simulink model "Scenario_13_CoDeSys"  (R2012b)
settings: Solver=ode3  StartTime=0.0  StopTime=inf  FixedStep=Sample_Time_Model  RelTol=1e-3
PreLoadFcn:
  | Variablen_Scenario13
InitFcn:
  | BT = randperm(9);
values from neighbouring files (symbols this model uses):
  Band_Geschwindigkeit = 1.47    [Variablen_Scenario13.m]
  Band_Sensor_Hell_2_Z = -6.5    [Variablen_Scenario13.m]
  Band_Sensor_Hell_3_Z = -10.36    [Variablen_Scenario13.m]
  Band_Sensor_Hell_4_Z = -14.64    [Variablen_Scenario13.m]
  Band_Sensor_Tolerance_Z = 0.2    [Variablen_Scenario13.m]
  Bauteil_Fallgeschwindigkeit = 0.4    [Variablen_Scenario13.m]
  Bauteil_Farbe_Metall = [0.8 0.8 0.8]    [Variablen_Scenario13.m]
  Bauteil_Farbe_Schwarz = [0.2 0.2 0.2]    [Variablen_Scenario13.m]
  Bauteil_Farbe_Weiss = [1 1 0.2]    [Variablen_Scenario13.m]
  Kran_Dauer_90_Grad = 5    [Variablen_Scenario13.m]
  Kran_Drehwinkel_90_Grad = 8050    [Variablen_Scenario13.m]
  Kran_Sensor_Position_Delta = 0.07    [Variablen_Scenario13.m]
  Sample_Time_Model = 0.05    [Variablen_Scenario13.m]
  Sample_Time_Simulation = 0.1    [Variablen_Scenario13.m]
  Sensor_Band_Metall_1 = -6.5    [Variablen_Scenario13.m]
  Sensor_Band_Metall_2 = -10.36    [Variablen_Scenario13.m]
libraries: simulink x557, vrlib x13, opclib x7, rtwinlib x1
(part 8 of 10)

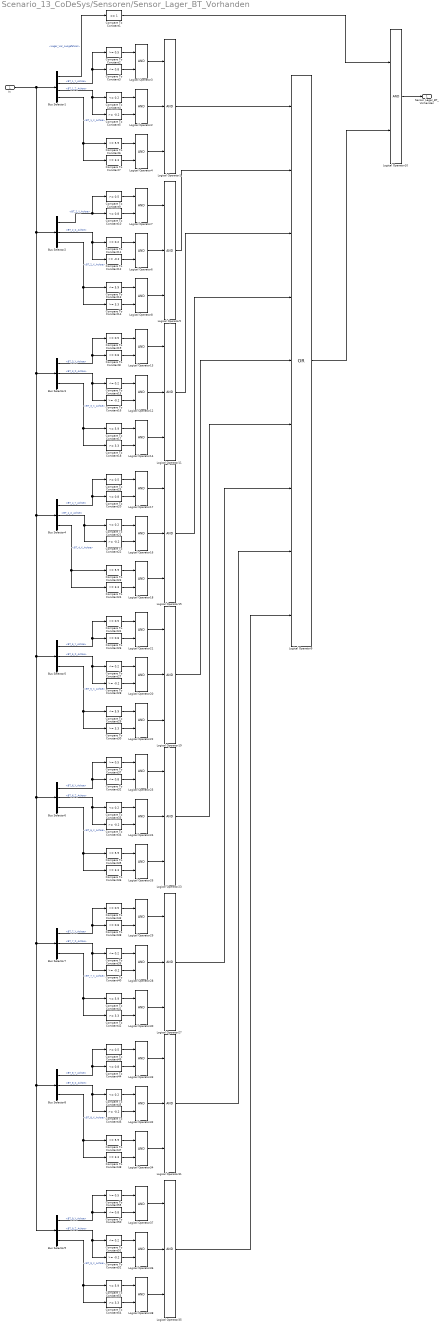
== system Scenario_13_CoDeSys/Sensoren/Sensor_Lager_BT_Vorhanden ==
  In : Inport
  Bus Selector1 : BusSelector  OutputSignals=Bauteil.Stempelanlage_BT.Stempelanlage.Lager.Lager_Ver_Ausgefahren,Bauteil.Stempelanlage_BT.Bauteil_1.BT_1_Y_Achse,Bauteil.Stempelanlage_BT.Bauteil_1.BT_1_Z_Achse,Bauteil.Stempelanlage_BT.Bauteil_1.BT_1_X_Achse
  Bus Selector2 : BusSelector  OutputSignals=Bauteil.Stempelanlage_BT.Bauteil_2.BT_2_Y_Achse,Bauteil.Stempelanlage_BT.Bauteil_2.BT_2_Z_Achse,Bauteil.Stempelanlage_BT.Bauteil_2.BT_2_X_Achse
  Bus Selector3 : BusSelector  OutputSignals=Bauteil.Stempelanlage_BT.Bauteil_3.BT_3_Y_Achse,Bauteil.Stempelanlage_BT.Bauteil_3.BT_3_Z_Achse,Bauteil.Stempelanlage_BT.Bauteil_3.BT_3_X_Achse
  Bus Selector4 : BusSelector  OutputSignals=Bauteil.Stempelanlage_BT.Bauteil_4.BT_4_Y_Achse,Bauteil.Stempelanlage_BT.Bauteil_4.BT_4_Z_Achse,Bauteil.Stempelanlage_BT.Bauteil_4.BT_4_X_Achse
  Bus Selector5 : BusSelector  OutputSignals=Bauteil.Stempelanlage_BT.Bauteil_5.BT_5_Y_Achse,Bauteil.Stempelanlage_BT.Bauteil_5.BT_5_Z_Achse,Bauteil.Stempelanlage_BT.Bauteil_5.BT_5_X_Achse
  Bus Selector6 : BusSelector  OutputSignals=Bauteil.Stempelanlage_BT.Bauteil_6.BT_6_Y_Achse,Bauteil.Stempelanlage_BT.Bauteil_6.BT_6_Z_Achse,Bauteil.Stempelanlage_BT.Bauteil_6.BT_6_X_Achse
  Bus Selector7 : BusSelector  OutputSignals=Bauteil.Stempelanlage_BT.Bauteil_7.BT_7_Y_Achse,Bauteil.Stempelanlage_BT.Bauteil_7.BT_7_Z_Achse,Bauteil.Stempelanlage_BT.Bauteil_7.BT_7_X_Achse
  Bus Selector8 : BusSelector  OutputSignals=Bauteil.Stempelanlage_BT.Bauteil_8.BT_8_Y_Achse,Bauteil.Stempelanlage_BT.Bauteil_8.BT_8_Z_Achse,Bauteil.Stempelanlage_BT.Bauteil_8.BT_8_X_Achse
  Bus Selector9 : BusSelector  OutputSignals=Bauteil.Stempelanlage_BT.Bauteil_9.BT_9_Y_Achse,Bauteil.Stempelanlage_BT.Bauteil_9.BT_9_Z_Achse,Bauteil.Stempelanlage_BT.Bauteil_9.BT_9_X_Achse
  Compare To Constant1 : simulink/Logic and Bit Operations/Compare To Constant  relop===  const=1  OutDataTypeStr=boolean
  Compare To Constant{3,8,10,20,26,32,38,44,50} (9 alike) : simulink/Logic and Bit Operations/Compare To Constant  relop=<=  const=0.8  OutDataTypeStr=boolean
  Compare To Constant{4,11,15,21,27,33,39,45,51} (9 alike) : simulink/Logic and Bit Operations/Compare To Constant  relop=<=  const=0.2  OutDataTypeStr=boolean
  Compare To Constant{5,12,16,22,28,34,40,46,52} (9 alike) : simulink/Logic and Bit Operations/Compare To Constant  relop=>=  const=-0.2  OutDataTypeStr=boolean
  Compare To Constant{6,13,17,23,29,35,41,47,53} (9 alike) : simulink/Logic and Bit Operations/Compare To Constant  relop=<=  const=5.9  OutDataTypeStr=boolean
  Compare To Constant{7,14,18,24,30,36,42,48,54} (9 alike) : simulink/Logic and Bit Operations/Compare To Constant  relop=>=  const=3.3  OutDataTypeStr=boolean
  Compare To Constant{2,9,19,25,31,37,43,49,55} (9 alike) : simulink/Logic and Bit Operations/Compare To Constant  relop=>=  const=0.5  OutDataTypeStr=boolean
  Logical Operator{1,5,11,15,19,23,27,31,35} (9 alike) : Logic  Inputs=3  AllPortsSameDT=off  OutDataTypeStr=boolean
  Logical Operator{2..4,6..8,10,12..14,16..18,20..22,24..26,28..30,32..34,36..38} (28 alike) : Logic  AllPortsSameDT=off  OutDataTypeStr=boolean
  Logical Operator9 : Logic  Operator=OR  Inputs=9  AllPortsSameDT=off  OutDataTypeStr=boolean
  Sensor_Lager_BT_Vorhanden : Outport
  wires:
  Compare To Constant2/1 -> Logical Operator3/1
  Compare To Constant3/1 -> Logical Operator3/2
  Compare To Constant1/1 -> Logical Operator10/1
  Logical Operator3/1 -> Logical Operator1/1
  Compare To Constant4/1 -> Logical Operator2/1
  Compare To Constant5/1 -> Logical Operator2/2
  Logical Operator2/1 -> Logical Operator1/2
  Compare To Constant6/1 -> Logical Operator4/1
  Compare To Constant7/1 -> Logical Operator4/2
  Logical Operator4/1 -> Logical Operator1/3
  Bus Selector1/1 -> Compare To Constant1/1  "<Lager_Ver_Ausgefahren>"
  Bus Selector1/2 -> Compare To Constant2/1, Compare To Constant3/1  "<BT_1_Y_Achse>"
  Bus Selector1/3 -> Compare To Constant4/1, Compare To Constant5/1  "<BT_1_Z_Achse>"
  Bus Selector1/4 -> Compare To Constant6/1, Compare To Constant7/1  "<BT_1_X_Achse>"
  Compare To Constant9/1 -> Logical Operator7/1
  Compare To Constant10/1 -> Logical Operator7/2
  Logical Operator7/1 -> Logical Operator5/1
  Logical Operator5/1 -> Logical Operator9/2
  Compare To Constant11/1 -> Logical Operator6/1
  Compare To Constant12/1 -> Logical Operator6/2
  Logical Operator6/1 -> Logical Operator5/2
  Compare To Constant13/1 -> Logical Operator8/1
  Compare To Constant14/1 -> Logical Operator8/2
  Logical Operator8/1 -> Logical Operator5/3
  Bus Selector2/1 -> Compare To Constant9/1, Compare To Constant10/1  "<BT_2_Y_Achse>"
  Bus Selector2/2 -> Compare To Constant11/1, Compare To Constant12/1  "<BT_2_Z_Achse>"
  Bus Selector2/3 -> Compare To Constant13/1, Compare To Constant14/1  "<BT_2_X_Achse>"
  Logical Operator9/1 -> Logical Operator10/2
  Logical Operator10/1 -> Sensor_Lager_BT_Vorhanden/1
  Logical Operator1/1 -> Logical Operator9/1
  Compare To Constant19/1 -> Logical Operator13/1
  Compare To Constant8/1 -> Logical Operator13/2
  Logical Operator13/1 -> Logical Operator11/1
  Compare To Constant15/1 -> Logical Operator12/1
  Compare To Constant16/1 -> Logical Operator12/2
  Logical Operator12/1 -> Logical Operator11/2
  Compare To Constant17/1 -> Logical Operator14/1
  Compare To Constant18/1 -> Logical Operator14/2
  Logical Operator14/1 -> Logical Operator11/3
  Bus Selector3/1 -> Compare To Constant19/1, Compare To Constant8/1  "<BT_3_Y_Achse>"
  Bus Selector3/2 -> Compare To Constant15/1, Compare To Constant16/1  "<BT_3_Z_Achse>"
  Bus Selector3/3 -> Compare To Constant17/1, Compare To Constant18/1  "<BT_3_X_Achse>"
  Compare To Constant25/1 -> Logical Operator17/1
  Compare To Constant20/1 -> Logical Operator17/2
  Logical Operator17/1 -> Logical Operator15/1
  Compare To Constant21/1 -> Logical Operator16/1
  Compare To Constant22/1 -> Logical Operator16/2
  Logical Operator16/1 -> Logical Operator15/2
  Compare To Constant23/1 -> Logical Operator18/1
  Compare To Constant24/1 -> Logical Operator18/2
  Logical Operator18/1 -> Logical Operator15/3
  Bus Selector4/1 -> Compare To Constant25/1, Compare To Constant20/1  "<BT_4_Y_Achse>"
  Compare To Constant31/1 -> Logical Operator21/1
  Compare To Constant26/1 -> Logical Operator21/2
  Logical Operator21/1 -> Logical Operator19/1
  Compare To Constant27/1 -> Logical Operator20/1
  Compare To Constant28/1 -> Logical Operator20/2
  Logical Operator20/1 -> Logical Operator19/2
  Compare To Constant29/1 -> Logical Operator22/1
  Compare To Constant30/1 -> Logical Operator22/2
  Logical Operator22/1 -> Logical Operator19/3
  Bus Selector5/1 -> Compare To Constant31/1, Compare To Constant26/1  "<BT_5_Y_Achse>"
  Bus Selector5/2 -> Compare To Constant27/1, Compare To Constant28/1  "<BT_5_Z_Achse>"
  Bus Selector5/3 -> Compare To Constant29/1, Compare To Constant30/1  "<BT_5_X_Achse>"
  Compare To Constant37/1 -> Logical Operator25/1
  Compare To Constant32/1 -> Logical Operator25/2
  Logical Operator25/1 -> Logical Operator23/1
  Compare To Constant33/1 -> Logical Operator24/1
  Compare To Constant34/1 -> Logical Operator24/2
  Logical Operator24/1 -> Logical Operator23/2
  Compare To Constant35/1 -> Logical Operator26/1
  Compare To Constant36/1 -> Logical Operator26/2
  Logical Operator26/1 -> Logical Operator23/3
  Bus Selector6/1 -> Compare To Constant37/1, Compare To Constant32/1  "<BT_6_Y_Achse>"
  Bus Selector6/2 -> Compare To Constant33/1, Compare To Constant34/1  "<BT_6_Z_Achse>"
  Bus Selector6/3 -> Compare To Constant35/1, Compare To Constant36/1  "<BT_6_X_Achse>"
  Logical Operator11/1 -> Logical Operator9/3
  Logical Operator15/1 -> Logical Operator9/4
  Logical Operator19/1 -> Logical Operator9/5
  Logical Operator23/1 -> Logical Operator9/6
  Bus Selector4/2 -> Compare To Constant21/1, Compare To Constant22/1  "<BT_4_Z_Achse>"
  Bus Selector4/3 -> Compare To Constant23/1, Compare To Constant24/1  "<BT_4_X_Achse>"
  Compare To Constant43/1 -> Logical Operator29/1
  Compare To Constant38/1 -> Logical Operator29/2
  Logical Operator29/1 -> Logical Operator27/1
  Compare To Constant39/1 -> Logical Operator28/1
  Compare To Constant40/1 -> Logical Operator28/2
  Logical Operator28/1 -> Logical Operator27/2
  Compare To Constant41/1 -> Logical Operator30/1
  Compare To Constant42/1 -> Logical Operator30/2
  Logical Operator30/1 -> Logical Operator27/3
  Bus Selector7/1 -> Compare To Constant43/1, Compare To Constant38/1  "<BT_7_Y_Achse>"
  Bus Selector7/2 -> Compare To Constant39/1, Compare To Constant40/1  "<BT_7_Z_Achse>"
  Bus Selector7/3 -> Compare To Constant41/1, Compare To Constant42/1  "<BT_7_X_Achse>"
  Compare To Constant49/1 -> Logical Operator33/1
  Compare To Constant44/1 -> Logical Operator33/2
  Logical Operator33/1 -> Logical Operator31/1
  Compare To Constant45/1 -> Logical Operator32/1
  Compare To Constant46/1 -> Logical Operator32/2
  Logical Operator32/1 -> Logical Operator31/2
  Compare To Constant47/1 -> Logical Operator34/1
  Compare To Constant48/1 -> Logical Operator34/2
  Logical Operator34/1 -> Logical Operator31/3
  Bus Selector8/1 -> Compare To Constant49/1, Compare To Constant44/1  "<BT_8_Y_Achse>"
  Bus Selector8/2 -> Compare To Constant45/1, Compare To Constant46/1  "<BT_8_Z_Achse>"
  Bus Selector8/3 -> Compare To Constant47/1, Compare To Constant48/1  "<BT_8_X_Achse>"
  Compare To Constant55/1 -> Logical Operator37/1
  Compare To Constant50/1 -> Logical Operator37/2
  Logical Operator37/1 -> Logical Operator35/1
  Compare To Constant51/1 -> Logical Operator36/1
  Compare To Constant52/1 -> Logical Operator36/2
  Logical Operator36/1 -> Logical Operator35/2
  Compare To Constant53/1 -> Logical Operator38/1
  Compare To Constant54/1 -> Logical Operator38/2
  Logical Operator38/1 -> Logical Operator35/3
  In/1 -> Bus Selector2/1, Bus Selector4/1, Bus Selector6/1, Bus Selector9/1, Bus Selector8/1, Bus Selector7/1, Bus Selector5/1, Bus Selector3/1, Bus Selector1/1
  Bus Selector9/1 -> Compare To Constant55/1, Compare To Constant50/1  "<BT_9_Y_Achse>"
  Bus Selector9/2 -> Compare To Constant51/1, Compare To Constant52/1  "<BT_9_Z_Achse>"
  Bus Selector9/3 -> Compare To Constant53/1, Compare To Constant54/1  "<BT_9_X_Achse>"
  Logical Operator35/1 -> Logical Operator9/9
  Logical Operator31/1 -> Logical Operator9/8
  Logical Operator27/1 -> Logical Operator9/7

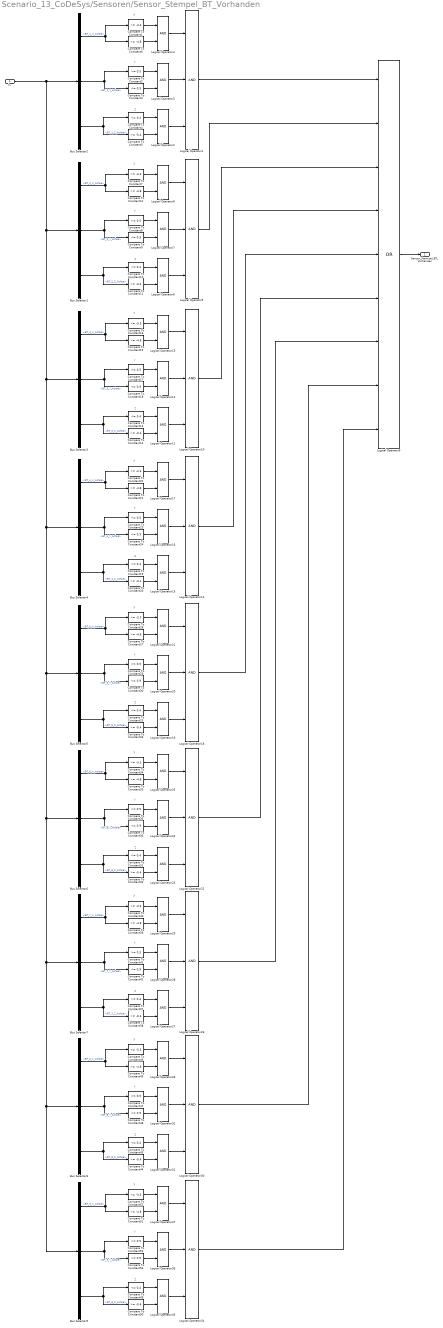
== system Scenario_13_CoDeSys/Sensoren/Sensor_Stempel_BT_Vorhanden ==
  note: Z
  note: Y
  note: X
  note: Z
  note: Y
  note: X
  note: Z
  note: Y
  note: X
  note: Z
  note: Y
  note: X
  note: Z
  note: Y
  note: X
  note: Z
  note: Y
  note: X
  note: Z
  note: Y
  note: X
  note: Z
  note: Y
  note: X
  note: Z
  note: Y
  note: X
  In : Inport
  Bus Selector1 : BusSelector  OutputSignals=Bauteil.Stempelanlage_BT.Bauteil_2.BT_2_X_Achse,Bauteil.Stempelanlage_BT.Bauteil_2.BT_2_Y_Achse,Bauteil.Stempelanlage_BT.Bauteil_2.BT_2_Z_Achse
  Bus Selector2 : BusSelector  OutputSignals=Bauteil.Stempelanlage_BT.Bauteil_1.BT_1_X_Achse,Bauteil.Stempelanlage_BT.Bauteil_1.BT_1_Y_Achse,Bauteil.Stempelanlage_BT.Bauteil_1.BT_1_Z_Achse
  Bus Selector3 : BusSelector  OutputSignals=Bauteil.Stempelanlage_BT.Bauteil_3.BT_3_X_Achse,Bauteil.Stempelanlage_BT.Bauteil_3.BT_3_Y_Achse,Bauteil.Stempelanlage_BT.Bauteil_3.BT_3_Z_Achse
  Bus Selector4 : BusSelector  OutputSignals=Bauteil.Stempelanlage_BT.Bauteil_4.BT_4_X_Achse,Bauteil.Stempelanlage_BT.Bauteil_4.BT_4_Y_Achse,Bauteil.Stempelanlage_BT.Bauteil_4.BT_4_Z_Achse
  Bus Selector5 : BusSelector  OutputSignals=Bauteil.Stempelanlage_BT.Bauteil_5.BT_5_X_Achse,Bauteil.Stempelanlage_BT.Bauteil_5.BT_5_Y_Achse,Bauteil.Stempelanlage_BT.Bauteil_5.BT_5_Z_Achse
  Bus Selector6 : BusSelector  OutputSignals=Bauteil.Stempelanlage_BT.Bauteil_6.BT_6_X_Achse,Bauteil.Stempelanlage_BT.Bauteil_6.BT_6_Y_Achse,Bauteil.Stempelanlage_BT.Bauteil_6.BT_6_Z_Achse
  Bus Selector7 : BusSelector  OutputSignals=Bauteil.Stempelanlage_BT.Bauteil_7.BT_7_X_Achse,Bauteil.Stempelanlage_BT.Bauteil_7.BT_7_Y_Achse,Bauteil.Stempelanlage_BT.Bauteil_7.BT_7_Z_Achse
  Bus Selector8 : BusSelector  OutputSignals=Bauteil.Stempelanlage_BT.Bauteil_8.BT_8_X_Achse,Bauteil.Stempelanlage_BT.Bauteil_8.BT_8_Y_Achse,Bauteil.Stempelanlage_BT.Bauteil_8.BT_8_Z_Achse
  Bus Selector9 : BusSelector  OutputSignals=Bauteil.Stempelanlage_BT.Bauteil_9.BT_9_X_Achse,Bauteil.Stempelanlage_BT.Bauteil_9.BT_9_Y_Achse,Bauteil.Stempelanlage_BT.Bauteil_9.BT_9_Z_Achse
  Compare To Constant{1,7,16,22,28,34,40,46,52} (9 alike) : simulink/Logic and Bit Operations/Compare To Constant  relop=<=  const=-3.3  OutDataTypeStr=boolean
  Compare To Constant{4,10,13,19,25,31,37,43,49} (9 alike) : simulink/Logic and Bit Operations/Compare To Constant  relop=<=  const=0.4  OutDataTypeStr=boolean
  Compare To Constant{5,11,14,20,26,32,38,44,50} (9 alike) : simulink/Logic and Bit Operations/Compare To Constant  relop=>=  const=-0.4  OutDataTypeStr=boolean
  Compare To Constant{6,12,15,21,27,33,39,45,51} (9 alike) : simulink/Logic and Bit Operations/Compare To Constant  relop=>=  const=-4.8  OutDataTypeStr=boolean
  Compare To Constant{2,8,17,23,29,35,41,47,53} (9 alike) : simulink/Logic and Bit Operations/Compare To Constant  relop=>=  const=0.5  OutDataTypeStr=boolean
  Compare To Constant{3,9,18,24,30,36,42,48,54} (9 alike) : simulink/Logic and Bit Operations/Compare To Constant  relop=<=  const=0.9  OutDataTypeStr=boolean
  Logical Operator{1,5,10,14,18,22,26,30,34} (9 alike) : Logic  Inputs=3  AllPortsSameDT=off  OutDataTypeStr=boolean
  Logical Operator{2..4,6..8,11..13,15..17,19..21,23..25,27..29,31..33,35..37} (27 alike) : Logic  AllPortsSameDT=off  OutDataTypeStr=boolean
  Logical Operator9 : Logic  Operator=OR  Inputs=9  AllPortsSameDT=off  OutDataTypeStr=boolean
  Sensor_Stempel_BT_Vorhanden : Outport
  wires:
  Compare To Constant2/1 -> Logical Operator3/1
  Compare To Constant3/1 -> Logical Operator3/2
  Logical Operator3/1 -> Logical Operator1/2
  Compare To Constant4/1 -> Logical Operator2/1
  Compare To Constant5/1 -> Logical Operator2/2
  Logical Operator2/1 -> Logical Operator1/3
  Compare To Constant1/1 -> Logical Operator4/1
  Compare To Constant6/1 -> Logical Operator4/2
  Logical Operator4/1 -> Logical Operator1/1
  Bus Selector2/1 -> Compare To Constant6/1, Compare To Constant1/1  "<BT_1_X_Achse>"
  Bus Selector2/2 -> Compare To Constant3/1, Compare To Constant2/1  "<BT_1_Y_Achse>"
  Bus Selector2/3 -> Compare To Constant5/1, Compare To Constant4/1  "<BT_1_Z_Achse>"
  Compare To Constant8/1 -> Logical Operator7/1
  Compare To Constant9/1 -> Logical Operator7/2
  Logical Operator7/1 -> Logical Operator5/2
  Compare To Constant10/1 -> Logical Operator6/1
  Compare To Constant11/1 -> Logical Operator6/2
  Logical Operator6/1 -> Logical Operator5/3
  Compare To Constant7/1 -> Logical Operator8/1
  Compare To Constant12/1 -> Logical Operator8/2
  Logical Operator8/1 -> Logical Operator5/1
  Bus Selector1/1 -> Compare To Constant12/1, Compare To Constant7/1  "<BT_2_X_Achse>"
  Bus Selector1/2 -> Compare To Constant9/1, Compare To Constant8/1  "<BT_2_Y_Achse>"
  Bus Selector1/3 -> Compare To Constant11/1, Compare To Constant10/1  "<BT_2_Z_Achse>"
  Logical Operator1/1 -> Logical Operator9/1
  Logical Operator5/1 -> Logical Operator9/2
  Logical Operator9/1 -> Sensor_Stempel_BT_Vorhanden/1
  Compare To Constant17/1 -> Logical Operator12/1
  Compare To Constant18/1 -> Logical Operator12/2
  Logical Operator12/1 -> Logical Operator10/2
  Compare To Constant13/1 -> Logical Operator11/1
  Compare To Constant14/1 -> Logical Operator11/2
  Logical Operator11/1 -> Logical Operator10/3
  Compare To Constant16/1 -> Logical Operator13/1
  Compare To Constant15/1 -> Logical Operator13/2
  Logical Operator13/1 -> Logical Operator10/1
  Bus Selector3/1 -> Compare To Constant15/1, Compare To Constant16/1  "<BT_3_X_Achse>"
  Bus Selector3/2 -> Compare To Constant18/1, Compare To Constant17/1  "<BT_3_Y_Achse>"
  Bus Selector3/3 -> Compare To Constant14/1, Compare To Constant13/1  "<BT_3_Z_Achse>"
  Compare To Constant23/1 -> Logical Operator16/1
  Compare To Constant24/1 -> Logical Operator16/2
  Logical Operator16/1 -> Logical Operator14/2
  Compare To Constant19/1 -> Logical Operator15/1
  Compare To Constant20/1 -> Logical Operator15/2
  Logical Operator15/1 -> Logical Operator14/3
  Compare To Constant22/1 -> Logical Operator17/1
  Compare To Constant21/1 -> Logical Operator17/2
  Logical Operator17/1 -> Logical Operator14/1
  Bus Selector4/1 -> Compare To Constant21/1, Compare To Constant22/1  "<BT_4_X_Achse>"
  Bus Selector4/2 -> Compare To Constant24/1, Compare To Constant23/1  "<BT_4_Y_Achse>"
  Bus Selector4/3 -> Compare To Constant20/1, Compare To Constant19/1  "<BT_4_Z_Achse>"
  Compare To Constant29/1 -> Logical Operator20/1
  Compare To Constant30/1 -> Logical Operator20/2
  Logical Operator20/1 -> Logical Operator18/2
  Compare To Constant25/1 -> Logical Operator19/1
  Compare To Constant26/1 -> Logical Operator19/2
  Logical Operator19/1 -> Logical Operator18/3
  Compare To Constant28/1 -> Logical Operator21/1
  Compare To Constant27/1 -> Logical Operator21/2
  Logical Operator21/1 -> Logical Operator18/1
  Bus Selector5/1 -> Compare To Constant27/1, Compare To Constant28/1  "<BT_5_X_Achse>"
  Bus Selector5/2 -> Compare To Constant30/1, Compare To Constant29/1  "<BT_5_Y_Achse>"
  Bus Selector5/3 -> Compare To Constant26/1, Compare To Constant25/1  "<BT_5_Z_Achse>"
  Compare To Constant35/1 -> Logical Operator24/1
  Compare To Constant36/1 -> Logical Operator24/2
  Logical Operator24/1 -> Logical Operator22/2
  Compare To Constant31/1 -> Logical Operator23/1
  Compare To Constant32/1 -> Logical Operator23/2
  Logical Operator23/1 -> Logical Operator22/3
  Compare To Constant34/1 -> Logical Operator25/1
  Compare To Constant33/1 -> Logical Operator25/2
  Logical Operator25/1 -> Logical Operator22/1
  Bus Selector6/1 -> Compare To Constant33/1, Compare To Constant34/1  "<BT_6_X_Achse>"
  Bus Selector6/2 -> Compare To Constant36/1, Compare To Constant35/1  "<BT_6_Y_Achse>"
  Bus Selector6/3 -> Compare To Constant32/1, Compare To Constant31/1  "<BT_6_Z_Achse>"
  Logical Operator10/1 -> Logical Operator9/3
  Logical Operator14/1 -> Logical Operator9/4
  Logical Operator18/1 -> Logical Operator9/5
  Logical Operator22/1 -> Logical Operator9/6
  Compare To Constant41/1 -> Logical Operator28/1
  Compare To Constant42/1 -> Logical Operator28/2
  Logical Operator28/1 -> Logical Operator26/2
  Compare To Constant37/1 -> Logical Operator27/1
  Compare To Constant38/1 -> Logical Operator27/2
  Logical Operator27/1 -> Logical Operator26/3
  Compare To Constant40/1 -> Logical Operator29/1
  Compare To Constant39/1 -> Logical Operator29/2
  Logical Operator29/1 -> Logical Operator26/1
  Bus Selector7/1 -> Compare To Constant39/1, Compare To Constant40/1  "<BT_7_X_Achse>"
  Bus Selector7/2 -> Compare To Constant42/1, Compare To Constant41/1  "<BT_7_Y_Achse>"
  Bus Selector7/3 -> Compare To Constant38/1, Compare To Constant37/1  "<BT_7_Z_Achse>"
  Compare To Constant47/1 -> Logical Operator32/1
  Compare To Constant48/1 -> Logical Operator32/2
  Logical Operator32/1 -> Logical Operator30/2
  Compare To Constant43/1 -> Logical Operator31/1
  Compare To Constant44/1 -> Logical Operator31/2
  Logical Operator31/1 -> Logical Operator30/3
  Compare To Constant46/1 -> Logical Operator33/1
  Compare To Constant45/1 -> Logical Operator33/2
  Logical Operator33/1 -> Logical Operator30/1
  Bus Selector8/1 -> Compare To Constant45/1, Compare To Constant46/1  "<BT_8_X_Achse>"
  Bus Selector8/2 -> Compare To Constant48/1, Compare To Constant47/1  "<BT_8_Y_Achse>"
  Bus Selector8/3 -> Compare To Constant44/1, Compare To Constant43/1  "<BT_8_Z_Achse>"
  Compare To Constant53/1 -> Logical Operator36/1
  Compare To Constant54/1 -> Logical Operator36/2
  Logical Operator36/1 -> Logical Operator34/2
  Compare To Constant49/1 -> Logical Operator35/1
  Compare To Constant50/1 -> Logical Operator35/2
  Logical Operator35/1 -> Logical Operator34/3
  Compare To Constant52/1 -> Logical Operator37/1
  Compare To Constant51/1 -> Logical Operator37/2
  Logical Operator37/1 -> Logical Operator34/1
  In/1 -> Bus Selector1/1, Bus Selector4/1, Bus Selector6/1, Bus Selector7/1, Bus Selector8/1, Bus Selector9/1, Bus Selector5/1, Bus Selector3/1, Bus Selector2/1
  Bus Selector9/1 -> Compare To Constant51/1, Compare To Constant52/1  "<BT_9_X_Achse>"
  Bus Selector9/2 -> Compare To Constant54/1, Compare To Constant53/1  "<BT_9_Y_Achse>"
  Bus Selector9/3 -> Compare To Constant50/1, Compare To Constant49/1  "<BT_9_Z_Achse>"
  Logical Operator26/1 -> Logical Operator9/7
  Logical Operator30/1 -> Logical Operator9/8
  Logical Operator34/1 -> Logical Operator9/9

== system Scenario_13_CoDeSys/Sensoren/Sensoren_Lager_Metall_und_Weiss_Schwarz ==
  In : Inport
  Bus Selector1 : BusSelector  OutputSignals=Eingaenge.Bauteile.BT_Eins,Bauteil.Stempelanlage_BT.Bauteil_1.BT_1_Bereit
  Bus Selector2 : BusSelector  OutputSignals=Eingaenge.Bauteile.BT_Zwei,Bauteil.Stempelanlage_BT.Bauteil_2.BT_2_Bereit
  Bus Selector3 : BusSelector  OutputSignals=Eingaenge.Bauteile.BT_Drei,Bauteil.Stempelanlage_BT.Bauteil_3.BT_3_Bereit
  Bus Selector4 : BusSelector  OutputSignals=Eingaenge.Bauteile.BT_Vier,Bauteil.Stempelanlage_BT.Bauteil_4.BT_4_Bereit
  Bus Selector5 : BusSelector  OutputSignals=Eingaenge.Bauteile.BT_Fuenf,Bauteil.Stempelanlage_BT.Bauteil_5.BT_5_Bereit
  Bus Selector6 : BusSelector  OutputSignals=Eingaenge.Bauteile.BT_Sechs,Bauteil.Stempelanlage_BT.Bauteil_6.BT_6_Bereit
  Bus Selector7 : BusSelector  OutputSignals=Eingaenge.Bauteile.BT_Sieben,Bauteil.Stempelanlage_BT.Bauteil_7.BT_7_Bereit
  Bus Selector8 : BusSelector  OutputSignals=Eingaenge.Bauteile.BT_Acht,Bauteil.Stempelanlage_BT.Bauteil_8.BT_8_Bereit
  Bus Selector9 : BusSelector  OutputSignals=Eingaenge.Bauteile.BT_Neun,Bauteil.Stempelanlage_BT.Bauteil_9.BT_9_Bereit
  Compare To Constant{,1,4,6,8,10,12,14,16} (9 alike) : simulink/Logic and Bit Operations/Compare To Constant  relop===  const=0  OutDataTypeStr=boolean
  Compare To Constant{2..3,5,7,9,11,13,15,17} (9 alike) : simulink/Logic and Bit Operations/Compare To Constant  relop===  const=2  OutDataTypeStr=boolean
  Constant{,1..8} (9 alike) : Constant  Value=3
  Logical Operator{,3..10} (9 alike) : Logic  Operator=OR  AllPortsSameDT=off  OutDataTypeStr=boolean
  Logical Operator1 : Logic  Operator=OR  Inputs=9  AllPortsSameDT=off  OutDataTypeStr=boolean
  Logical Operator2 : Logic  Operator=OR  Inputs=9  AllPortsSameDT=off  OutDataTypeStr=boolean
  Switch{,1..8} (9 alike) : Switch  Threshold=1
  Sensor_Lager_Metall : Outport
  Sensor_Lager_Helligkeit : Outport  Port=2
  wires:
  Compare To Constant2/1 -> Logical Operator2/1, Logical Operator/2
  Compare To Constant/1 -> Logical Operator/1
  Bus Selector1/1 -> Switch/1  "<BT_Eins>"
  Switch/1 -> Compare To Constant2/1, Compare To Constant/1
  Constant/1 -> Switch/3
  Logical Operator/1 -> Logical Operator1/1
  Compare To Constant3/1 -> Logical Operator2/2, Logical Operator3/2
  Compare To Constant1/1 -> Logical Operator3/1
  Switch1/1 -> Compare To Constant3/1, Compare To Constant1/1
  Constant1/1 -> Switch1/3
  Logical Operator3/1 -> Logical Operator1/2
  Compare To Constant5/1 -> Logical Operator2/3, Logical Operator4/2
  Compare To Constant4/1 -> Logical Operator4/1
  Switch2/1 -> Compare To Constant5/1, Compare To Constant4/1
  Constant2/1 -> Switch2/3
  Logical Operator4/1 -> Logical Operator1/3
  Compare To Constant7/1 -> Logical Operator2/4, Logical Operator5/2
  Compare To Constant6/1 -> Logical Operator5/1
  Switch3/1 -> Compare To Constant7/1, Compare To Constant6/1
  Constant3/1 -> Switch3/3
  Logical Operator5/1 -> Logical Operator1/4
  Compare To Constant9/1 -> Logical Operator2/5, Logical Operator6/2
  Compare To Constant8/1 -> Logical Operator6/1
  Switch4/1 -> Compare To Constant9/1, Compare To Constant8/1
  Constant4/1 -> Switch4/3
  Logical Operator6/1 -> Logical Operator1/5
  Compare To Constant11/1 -> Logical Operator2/6, Logical Operator7/2
  Compare To Constant10/1 -> Logical Operator7/1
  Switch5/1 -> Compare To Constant11/1, Compare To Constant10/1
  Constant5/1 -> Switch5/3
  Logical Operator7/1 -> Logical Operator1/6
  Logical Operator2/1 -> Sensor_Lager_Metall/1
  Logical Operator1/1 -> Sensor_Lager_Helligkeit/1
  Bus Selector1/2 -> Switch/2  "<BT_1_Bereit>"
  Bus Selector2/1 -> Switch1/1  "<BT_Zwei>"
  Bus Selector2/2 -> Switch1/2  "<BT_2_Bereit>"
  Bus Selector3/1 -> Switch2/1  "<BT_Drei>"
  Bus Selector3/2 -> Switch2/2  "<BT_3_Bereit>"
  Bus Selector4/1 -> Switch3/1  "<BT_Vier>"
  Bus Selector4/2 -> Switch3/2  "<BT_4_Bereit>"
  Bus Selector5/1 -> Switch4/1  "<BT_Fuenf>"
  Bus Selector5/2 -> Switch4/2  "<BT_5_Bereit>"
  Bus Selector6/1 -> Switch5/1  "<BT_Sechs>"
  Bus Selector6/2 -> Switch5/2  "<BT_6_Bereit>"
  Compare To Constant13/1 -> Logical Operator2/7, Logical Operator8/2
  Compare To Constant12/1 -> Logical Operator8/1
  Switch6/1 -> Compare To Constant13/1, Compare To Constant12/1
  Constant6/1 -> Switch6/3
  Logical Operator8/1 -> Logical Operator1/7
  Bus Selector7/1 -> Switch6/1  "<BT_Sieben>"
  Bus Selector7/2 -> Switch6/2  "<BT_7_Bereit>"
  Compare To Constant15/1 -> Logical Operator2/8, Logical Operator9/2
  Compare To Constant14/1 -> Logical Operator9/1
  Switch7/1 -> Compare To Constant15/1, Compare To Constant14/1
  Constant7/1 -> Switch7/3
  Logical Operator9/1 -> Logical Operator1/8
  Bus Selector8/1 -> Switch7/1  "<BT_Acht>"
  Bus Selector8/2 -> Switch7/2  "<BT_8_Bereit>"
  Compare To Constant17/1 -> Logical Operator2/9, Logical Operator10/2
  Compare To Constant16/1 -> Logical Operator10/1
  Switch8/1 -> Compare To Constant17/1, Compare To Constant16/1
  Constant8/1 -> Switch8/3
  Logical Operator10/1 -> Logical Operator1/9
  In/1 -> Bus Selector2/1, Bus Selector3/1, Bus Selector4/1, Bus Selector7/1, Bus Selector8/1, Bus Selector9/1, Bus Selector6/1, Bus Selector5/1, Bus Selector1/1
  Bus Selector9/1 -> Switch8/1  "<BT_Neun>"
  Bus Selector9/2 -> Switch8/2  "<BT_9_Bereit>"

== system Scenario_13_CoDeSys/Sensoren/Stempel_Druck_Ist ==
  Sensor_Stempel_BT_Vorhanden : Inport
  Stempel_Halterung_Eingefahren : Inport  Port=2
  Stempel_Zyl_Ausgefahren : Inport  Port=3
  Stempel_Druck_Soll : Inport  Port=4
  Constant : Constant  Value=0
  Logical Operator1 : Logic  Inputs=3  AllPortsSameDT=off  OutDataTypeStr=boolean
  Switch : Switch  Threshold=1
  Stempel_Druck_Ist : Outport
  wires:
  Stempel_Halterung_Eingefahren/1 -> Logical Operator1/2
  Sensor_Stempel_BT_Vorhanden/1 -> Logical Operator1/1
  Stempel_Zyl_Ausgefahren/1 -> Logical Operator1/3
  Logical Operator1/1 -> Switch/2
  Switch/1 -> Stempel_Druck_Ist/1
  Stempel_Druck_Soll/1 -> Switch/1
  Constant/1 -> Switch/3

== system Scenario_13_CoDeSys/Signal Expander/BT_Lager_Status ==
  BT_1_Lager_Position : Inport
  BT_2_Lager_Position : Inport  Port=2
  BT_3_Lager_Position : Inport  Port=3
  BT_4_Lager_Position : Inport  Port=4
  BT_5_Lager_Position : Inport  Port=5
  BT_6_Lager_Position : Inport  Port=6
  BT_7_Lager_Position : Inport  Port=7
  BT_8_Lager_Position : Inport  Port=8
  BT_9_Lager_Position : Inport  Port=9
  Add : Sum  Inputs=+++++++++
  Add1 : Sum  Inputs=+++++++++
  Add2 : Sum  Inputs=+++++++++
  Compare To Constant{1..2,5,8,11,14,17,20,23} (9 alike) : simulink/Logic and Bit Operations/Compare To Constant  relop===  const=1  OutDataTypeStr=boolean
  Compare To Constant{3,6,10,12,15,18,21,24,26} (9 alike) : simulink/Logic and Bit Operations/Compare To Constant  relop===  const=3  OutDataTypeStr=boolean
  Compare To Constant{4,7,9,13,16,19,22,25,27} (9 alike) : simulink/Logic and Bit Operations/Compare To Constant  relop===  const=2  OutDataTypeStr=boolean
  Lager_1_Status : Outport
  Lager_2_Status : Outport  Port=2
  Lager_3_Status : Outport  Port=3
  wires:
  BT_1_Lager_Position/1 -> Compare To Constant10/1, Compare To Constant9/1, Compare To Constant1/1
  BT_2_Lager_Position/1 -> Compare To Constant12/1, Compare To Constant13/1, Compare To Constant11/1
  BT_3_Lager_Position/1 -> Compare To Constant15/1, Compare To Constant16/1, Compare To Constant14/1
  BT_4_Lager_Position/1 -> Compare To Constant18/1, Compare To Constant19/1, Compare To Constant17/1
  BT_5_Lager_Position/1 -> Compare To Constant21/1, Compare To Constant22/1, Compare To Constant20/1
  BT_6_Lager_Position/1 -> Compare To Constant24/1, Compare To Constant25/1, Compare To Constant23/1
  Compare To Constant1/1 -> Add/1
  Compare To Constant11/1 -> Add/2
  Compare To Constant14/1 -> Add/3
  Compare To Constant17/1 -> Add/4
  Compare To Constant20/1 -> Add/5
  Compare To Constant23/1 -> Add/6
  Compare To Constant9/1 -> Add1/1
  Compare To Constant13/1 -> Add1/2
  Compare To Constant16/1 -> Add1/3
  Compare To Constant19/1 -> Add1/4
  Compare To Constant22/1 -> Add1/5
  Compare To Constant25/1 -> Add1/6
  Compare To Constant24/1 -> Add2/6
  Compare To Constant21/1 -> Add2/5
  Compare To Constant18/1 -> Add2/4
  Compare To Constant15/1 -> Add2/3
  Compare To Constant12/1 -> Add2/2
  Compare To Constant10/1 -> Add2/1
  Add/1 -> Lager_1_Status/1
  Add1/1 -> Lager_2_Status/1
  Add2/1 -> Lager_3_Status/1
  BT_7_Lager_Position/1 -> Compare To Constant3/1, Compare To Constant4/1, Compare To Constant2/1
  BT_8_Lager_Position/1 -> Compare To Constant6/1, Compare To Constant7/1, Compare To Constant5/1
  BT_9_Lager_Position/1 -> Compare To Constant26/1, Compare To Constant27/1, Compare To Constant8/1
  Compare To Constant2/1 -> Add/7
  Compare To Constant5/1 -> Add/8
  Compare To Constant8/1 -> Add/9
  Compare To Constant4/1 -> Add1/7
  Compare To Constant7/1 -> Add1/8
  Compare To Constant27/1 -> Add1/9
  Compare To Constant3/1 -> Add2/7
  Compare To Constant6/1 -> Add2/8
  Compare To Constant26/1 -> Add2/9

== system Scenario_13_CoDeSys/Signal Expander/Berechne Band Geschwindigkeit ==
  Constant : Constant  Value=Band_Geschwindigkeit
  Multi : Product  Inputs=**
  Sample_Time : Constant  Value=Sample_Time_Model
  Band_Geschwindigkeit : Outport
  wires:
  Sample_Time/1 -> Multi/2
  Constant/1 -> Multi/1
  Multi/1 -> Band_Geschwindigkeit/1

== system Scenario_13_CoDeSys/Signal Expander/Kran_Position_Sensor ==
  In : Inport
  Abs : Abs
  Add : Sum
  Add1 : Sum  Inputs=+-
  Add2 : Sum
  Add3 : Sum  Inputs=+-
  Constant{,1,3..4,6} (5 alike) : Constant  Value=Kran_Sensor_Position_Delta
  Constant2 : Constant  Value=3.1416
  Constant5 : Constant  Value=1.5708
  Logical Operator1 : Logic  AllPortsSameDT=off  OutDataTypeStr=boolean
  Logical Operator2 : Logic  AllPortsSameDT=off  OutDataTypeStr=boolean
  Relational Operator : RelationalOperator  OutDataTypeStr=boolean
  Relational Operator{1..4} (4 alike) : RelationalOperator  Operator=<=  OutDataTypeStr=boolean
  Sensor_Kran_Stellung_Lager : Outport
  Sensor_Kran_Stellung_Band : Outport  Port=2
  Sensor_Kran_Stellung_Stempel : Outport  Port=3
  wires:
  Constant/1 -> Relational Operator/1
  Abs/1 -> Relational Operator/2
  Relational Operator/1 -> Sensor_Kran_Stellung_Lager/1
  Constant1/1 -> Add/1
  Constant2/1 -> Add1/1, Add/2
  Constant3/1 -> Add1/2
  Add/1 -> Relational Operator1/2
  Add1/1 -> Relational Operator2/1
  Relational Operator1/1 -> Logical Operator1/1
  Relational Operator2/1 -> Logical Operator1/2
  Logical Operator1/1 -> Sensor_Kran_Stellung_Stempel/1
  In/1 -> Relational Operator4/2, Relational Operator3/1, Relational Operator2/2, Relational Operator1/1, Abs/1
  Constant4/1 -> Add2/1
  Constant5/1 -> Add3/1, Add2/2
  Constant6/1 -> Add3/2
  Add2/1 -> Relational Operator3/2
  Add3/1 -> Relational Operator4/1
  Relational Operator3/1 -> Logical Operator2/1
  Relational Operator4/1 -> Logical Operator2/2
  Logical Operator2/1 -> Sensor_Kran_Stellung_Band/1

== system Scenario_13_CoDeSys/Signal Expander/Subsystem ==
  Notaus_Knopf : Inport
  BT_Y_In : Inport  Port=2
  BT_Lager_In : Inport  Port=3
  BT_angesaugt_in : Inport  Port=4
  BT_Bereit : Inport  Port=5
  Add : Sum  Inputs=-+
  Compare To Constant : simulink/Logic and Bit Operations/Compare To Constant  relop===  const=0  OutDataTypeStr=boolean
  Constant : Constant  Value=5000
  Constant1 : Constant  Value=0
  Constant2 : Constant  Value=0
  Constant3 : Constant  Value=0
  Detect Decrease : simulink/Logic and Bit Operations/Detect Decrease  vinit=0.0  InputProcessing=Inherited  OutDataTypeStr=boolean
  Logical Operator : Logic  Operator=OR  AllPortsSameDT=off  OutDataTypeStr=boolean
  Logical Operator1 : Logic  Inputs=3  AllPortsSameDT=off  OutDataTypeStr=boolean
  Logical Operator2 : Logic  Operator=OR  AllPortsSameDT=off  OutDataTypeStr=boolean
  Memory : Memory
  Memory1 : Memory
  Switch{,1..3} (4 alike) : Switch  Threshold=1
  BT_Y_Out : Outport
  BT_Angesaugt_Out : Outport  Port=2
  BT_Lager_Out : Outport  Port=3
  BT_Bereit_Out : Outport  Port=4
  wires:
  BT_Bereit/1 -> Switch3/3, Logical Operator/1
  Memory/1 -> Logical Operator/2
  BT_Y_In/1 -> Switch/3, Add/2
  Compare To Constant/1 -> Logical Operator1/1
  Logical Operator/1 -> Memory/1, Logical Operator1/2
  Constant/1 -> Add/1
  Add/1 -> Switch/1
  Switch/1 -> BT_Y_Out/1
  Notaus_Knopf/1 -> Detect Decrease/1
  Detect Decrease/1 -> Logical Operator1/3
  Logical Operator1/1 -> Logical Operator2/1
  Memory1/1 -> Logical Operator2/2
  Logical Operator2/1 -> Switch1/2, Switch3/2, Switch2/2, Switch/2, Memory1/1
  BT_angesaugt_in/1 -> Switch1/3
  Constant1/1 -> Switch1/1
  Switch1/1 -> BT_Angesaugt_Out/1
  BT_Lager_In/1 -> Switch2/3, Compare To Constant/1
  Constant2/1 -> Switch2/1
  Switch2/1 -> BT_Lager_Out/1
  Constant3/1 -> Switch3/1
  Switch3/1 -> BT_Bereit_Out/1

== stateflow chart Scenario_13_CoDeSys/Signal Expander/Band_Zyl_2 ==
  state Schrittgroesse [function]
    (default) -> (junction 166) : {Schrittgroesse = (3* Sample_Time)/0.11}
  state Berechne_Naechste_Position_Einfahren [function]
    (default) -> (junction 156) : {Naechste_Position = Zyl_2_X_Achse - Schrittgroesse;}
    (junction 156) -> (junction 157) [order 1] : [Naechste_Position <= -1]
    (junction 156) -> (junction 158) [order 2] : {Zyl_2_X_Achse = Naechste_Position;}
    (junction 157) -> (junction 159) : {Zyl_2_X_Achse = -1;}
    (junction 159) -> (junction 158)
  state Zyl_2_Bereit
    entry: Zyl_2_X_Achse = -1;
    Band_Zyl_2_Eingefahren = 1;
    exit: Band_Zyl_2_Eingefahren = 0;
  state Berechne_Naechste_Position_Ausfahren [function]
    (default) -> (junction 146) : {Naechste_Position = Zyl_2_X_Achse + Schrittgroesse;}
    (junction 146) -> (junction 147) [order 1] : [Naechste_Position >= 2]
    (junction 146) -> (junction 148) [order 2] : {Zyl_2_X_Achse = Naechste_Position;}
    (junction 147) -> (junction 149) : {Zyl_2_X_Achse = 2;}
    (junction 149) -> (junction 148)
  state r = Stop_Einfahren [function]
    (default) -> (junction 181) : {r=0}
    (junction 181) -> (junction 182) [order 1] : [!Zyl_2_Einfahren || (Zyl_2_Ausfahren && Zyl_2_Einfahren)]
    (junction 182) -> (junction 184) : {r=1}
    (junction 181) -> (junction 183) [order 2]
    (junction 184) -> (junction 183)
  state Stop
  state Zyl_2_Ausfahren
    during: Berechne_Naechste_Position_Ausfahren();
  state r = Stop_Ausfahren [function]
    (default) -> (junction 192) : {r=0}
    (junction 192) -> (junction 193) [order 1] : [!Zyl_2_Ausfahren || (Zyl_2_Ausfahren && Zyl_2_Einfahren)]
    (junction 193) -> (junction 195) : {r=1}
    (junction 192) -> (junction 194) [order 2]
    (junction 195) -> (junction 194)
  state r = Continue_Einfahren [function]
    (default) -> (junction 170) : {r=0}
    (junction 170) -> (junction 171) [order 1] : [Zyl_2_Einfahren && !Zyl_2_Ausfahren]
    (junction 171) -> (junction 173) : {r=1}
    (junction 170) -> (junction 172) [order 2]
    (junction 173) -> (junction 172)
  state Zyl_2_Ausgefahren
    entry: Band_Zyl_2_Ausgefahren = 1;
    Zyl_2_X_Achse = 2;
    exit: Band_Zyl_2_Ausgefahren = 0;
  state r = Continue_Ausfahren [function]
    (default) -> (junction 203) : {r=0}
    (junction 203) -> (junction 204) [order 1] : [Zyl_2_Ausfahren && !Zyl_2_Einfahren]
    (junction 204) -> (junction 206) : {r=1}
    (junction 203) -> (junction 205) [order 2]
    (junction 206) -> (junction 205)
  state Zyl_2_Einfahren
    during: Berechne_Naechste_Position_Einfahren();
  (default) -> Zyl_2_Bereit : {Schrittgroesse();}
  Zyl_2_Bereit -> Zyl_2_Ausfahren : [Zyl_2_Ausfahren && !Zyl_2_Einfahren]
  Zyl_2_Einfahren -> Zyl_2_Bereit [order 1] : [Zyl_2_X_Achse <= -1]
  Zyl_2_Ausfahren -> Stop [order 2] : [Stop_Ausfahren()]
  Stop -> Zyl_2_Ausfahren [order 1] : [Continue_Ausfahren()]
  Stop -> Zyl_2_Einfahren [order 2] : [Continue_Einfahren()]
  Zyl_2_Einfahren -> Stop [order 2] : [Stop_Einfahren()]
  Zyl_2_Ausfahren -> Zyl_2_Ausgefahren [order 1] : [Zyl_2_X_Achse >= 2]
  Zyl_2_Ausgefahren -> Zyl_2_Einfahren : [Zyl_2_Einfahren && !Zyl_2_Ausfahren]
  data: r function_output double; r function_output double; r function_output double; r function_output double; Zyl_2_Einfahren input; Schrittgroesse output double; Zyl_2_X_Achse output double; Zyl_2_Ausfahren input; Band_Zyl_2_Eingefahren output double; Band_Zyl_2_Ausgefahren output double; Sample_Time input; Naechste_Position local double
